simulink model "partB_ex3_projective"  (R2024b)
settings: Solver=FixedStepDiscrete  StartTime=0.0  StopTime=0  RelTol=1e-3  EnableMultiTasking=on
undefined symbols (not defined in the file or in its folder): gray
libraries: visionsources x1, visiongeotforms x1
settings Model: Creator=FxMain  LastModifiedBy=Nick
settings SolverCC: AlgebraicLoopSolver=TrustRegion
settings DataIOCC: LimitDataPoints=on  SaveFormat=Array  SignalLoggingSaveFormat=ModelDataLogs  ReturnWorkspaceOutputs=off
settings OptimizationCC: ExpressionDepthLimit=2147483647  LifeSpan=inf
settings DebuggingCC: UnderspecifiedInitializationDetection=Classic  MergeDetectMultiDrivingBlocksExec=none  SolverPrmCheckMsg=warning  FcnCallInpInsideContextMsg=warning  UnconnectedInputMsg=warning  UnconnectedOutputMsg=warning  UnconnectedLineMsg=warning  StateNameClashWarn=warning  SFUnexpectedBacktrackingDiag=warning  SFNoUnconditionalDefaultTransitionDiag=warning  SFExecutionAtInitializationDiag=none  ArithmeticOperatorsInVariantConditions=warning
settings HardwareCC: ProdBitPerPointer=32  ProdBitPerSizeT=32  ProdBitPerPtrDiffT=32  ProdLargestAtomicFloat=None  ProdIntDivRoundTo=Undefined  ProdEndianess=Unspecified  ProdWordSize=32  ProdHWDeviceType=32-bit Generic
settings ModelReferenceCC: EnableRefExpFcnMdlSchedulingChecks=on  PropagateSignalLabelsOutOfModel=off
settings SFSimCC: SimUseLocalCustomCode=off  CustomCodeUndefinedFunction=UseInterfaceOnly
settings RTWCC: RTWUseLocalCustomCode=off  GPUComputeCapability=3.5
settings CodeAppCC: StateflowObjectComments=on
settings GRTTargetCC: TargetLangStandard=C89/C90 (ANSI)  CombineOutputUpdateFcns=off  GRTInterface=on
settings ConfigComp: CovMetricSettings=dw  CovSaveCumulativeToWorkspaceVar=on  CovSaveSingleToWorkspaceVar=on  CovExternalEMLEnable=off

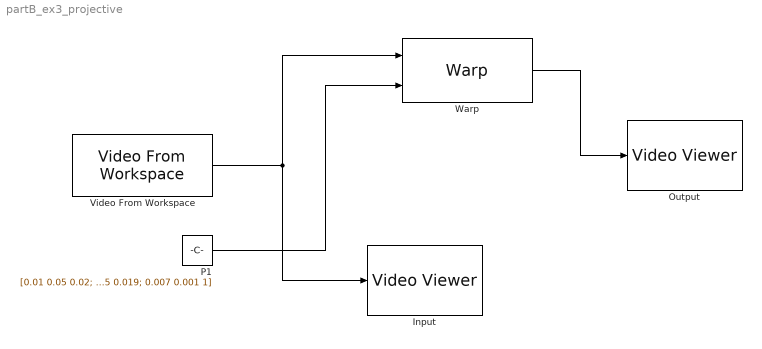
== system partB_ex3_projective ==
  Input : VideoViewer  colormapValue=gray(256)  FigPos=[2266 753 508 300]
  Output : VideoViewer  colormapValue=gray(256)  FigPos=[3066 747 575 402]
  P1 : Constant  Value=[0.01 0.05 0.02; 0.033 0.0325 0.019; 0.007 0.001 1]  VectorParams1D=off
      settings: SamplingMode=Frame based
  Video From Workspace : visionsources/Video From Workspace  signal=vid2  Ts=1  finalout=Obsolete  finaloutActive=Cyclic repetition  imagePorts=One multidimensional signal  OutPortLabels=R|G|B
  Warp : visiongeotforms/Warp  TransformMatrixSource=Input port  TransformMatrix=eye( 3 )  InterpolationMethod=Bilinear  BackgroundFillValue=0  OutputImagePositionSource=Custom  OutputImagePosition=[-100 -100 800 600]  ROIInputPort=off  ROIValidityOutputPort=off  SimulateUsing=Interpreted execution
  wires:
  Video From Workspace/1 -> Warp/1, Input/1
  Warp/1 -> Output/1
  P1/1 -> Warp/2
